simulink subsystem "PWM"  (R2020b)
settings: Solver=VariableStepAuto  StartTime=0.0  StopTime=10.0  RelTol=1e-3
libraries: fl_lib x46, ee_lib x14, nesl_utility x12
settings Model: Creator=marti  LastModifiedBy=marti

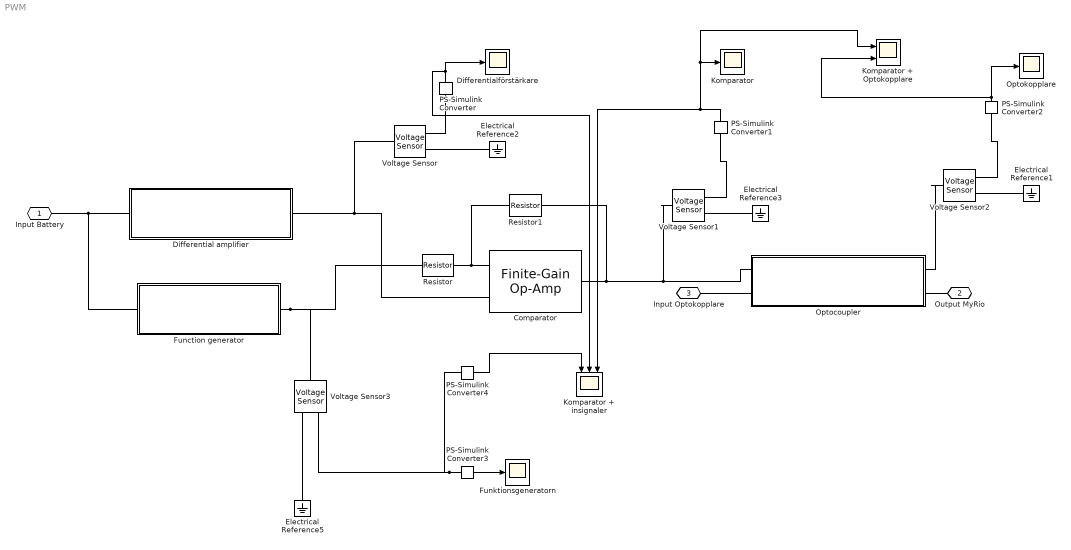
== system PWM ==
  Comparator : ee_lib/Integrated Circuits/Finite-Gain Op-Amp  A=1000  Rin=1e6 Ohm  Rout=0 Ohm  Vmin=0 V  Vmax=12.8 V  noise_mode=0  v_noise=30e-9 V/Hz^0.50000  noise_prm=1  i_noise=0.5e-12 A/Hz^0.50000  ip_noise=0.5e-12 A/Hz^0.50000  in_noise=0.5e-12 A/Hz^0.50000  sample_time=1e-3 s  repeatability=1  auto_seed_v=576828300  auto_seed_ip=423458404  auto_seed_in=610002388  user_seed_v=0  user_seed_ip=0  user_seed_in=0
      settings: SourceProductBaseCode=PS  InternalSimscapePortConfiguration="{\"Bottom\":[],\"Left\":[{\"id\":\"p\",\"label\":\"+\",\"type\":\"foundation.electrical.electrical\"},{\"id\":\"n\",\"label\":\"-\",\"type\":\"foundation.electrical.electrical\"}],\"Right\":[{\"id\":\"out\",\"label\":\"\",\"type\":\"foundation.electrical.electrical\"}],\"Top\":[]}"
  Differential amplifier : Subsystem
  Differentialförstärkare : Scope
  Electrical Reference{1..3,5} (4 alike) : fl_lib/Electrical/Electrical Elements/Electrical Reference
  Function generator : Subsystem
  Funktionsgeneratorn : Scope
  Komparator : Scope
  Komparator + Optokopplare : Scope  NumInputPorts=2
  Komparator + insignaler : Scope  NumInputPorts=3
  Optocoupler : Subsystem
  Optokopplare : Scope
  PS-Simulink Converter : nesl_utility/PS-Simulink Converter  PhysicalDomain=network_engine_domain  SubClassName=ps_output  LeftPortType=input  RightPortType=output  PseudoPeriodic=off  Frequencies=[]  Unit=inherit  AffineConversion=off
  PS-Simulink Converter1 : nesl_utility/PS-Simulink Converter  PhysicalDomain=network_engine_domain  SubClassName=ps_output  LeftPortType=input  RightPortType=output  PseudoPeriodic=off  Frequencies=[]  Unit=inherit  AffineConversion=off
  PS-Simulink Converter2 : nesl_utility/PS-Simulink Converter  PhysicalDomain=network_engine_domain  SubClassName=ps_output  LeftPortType=input  RightPortType=output  PseudoPeriodic=off  Frequencies=[]  Unit=inherit  AffineConversion=off
  PS-Simulink Converter3 : nesl_utility/PS-Simulink Converter  PhysicalDomain=network_engine_domain  SubClassName=ps_output  LeftPortType=input  RightPortType=output  PseudoPeriodic=off  Frequencies=[]  Unit=1  AffineConversion=off
  PS-Simulink Converter4 : nesl_utility/PS-Simulink Converter  PhysicalDomain=network_engine_domain  SubClassName=ps_output  LeftPortType=input  RightPortType=output  PseudoPeriodic=off  Frequencies=[]  Unit=1  AffineConversion=off
  Resistor : fl_lib/Electrical/Electrical Elements/Resistor  R=10000 Ohm  i_specify=off  i_priority=None  i=0 A  i_nominal_specify=off  i_nominal_unit=A  i_nominal_value=1  v_specify=off  v_priority=None  v=0 V  v_nominal_specify=off  v_nominal_unit=V  v_nominal_value=1
  Resistor1 : fl_lib/Electrical/Electrical Elements/Resistor  R=100000 Ohm  i_specify=off  i_priority=None  i=0 A  i_nominal_specify=off  i_nominal_unit=A  i_nominal_value=1  v_specify=off  v_priority=None  v=0 V  v_nominal_specify=off  v_nominal_unit=V  v_nominal_value=1
  Voltage Sensor{,1..3} (4 alike) : fl_lib/Electrical/Electrical Sensors/Voltage Sensor
      Voltage Sensor3 settings: SourceProductName=Foundation Library
      Voltage Sensor settings: LogSimulationData=on
  Input Battery : PMIOPort  Side=Left
  Output MyRio : PMIOPort  Port=2  Side=Right
  Input Optokopplare : PMIOPort  Port=3  Side=Left
  wires:
  PS-Simulink Converter/1 -> Komparator + insignaler/2, Differentialförstärkare/1
  PS-Simulink Converter3/1 -> Funktionsgeneratorn/1
  PS-Simulink Converter4/1 -> Komparator + insignaler/1
  PS-Simulink Converter2/1 -> Komparator + Optokopplare/2, Optokopplare/1
  PS-Simulink Converter1/1 -> Komparator/1, Komparator + Optokopplare/1, Komparator + insignaler/3
  connections:
  Function generator/LConn1 -- Input Battery/RConn1 -- Differential amplifier/LConn1
  PS-Simulink Converter3/LConn1 -- Voltage Sensor3/RConn1 -- PS-Simulink Converter4/LConn1
  Differential amplifier/RConn1 -- Voltage Sensor/LConn1 -- Comparator/LConn2
  Function generator/RConn1 -- Voltage Sensor3/LConn1 -- Resistor/LConn1
  Resistor1/RConn1 -- Comparator/RConn1 -- Voltage Sensor1/LConn1 -- Optocoupler/LConn1
  Resistor1/LConn1 -- Resistor/RConn1 -- Comparator/LConn1
  Input Optokopplare/RConn1 -- Optocoupler/LConn2
  Optocoupler/RConn2 -- Output MyRio/RConn1
  Voltage Sensor/RConn1 -- PS-Simulink Converter/LConn1
  Voltage Sensor3/RConn2 -- Electrical Reference5/LConn1
  Electrical Reference3/LConn1 -- Voltage Sensor1/RConn2
  Voltage Sensor2/LConn1 -- Optocoupler/RConn1
  PS-Simulink Converter1/LConn1 -- Voltage Sensor1/RConn1
  Voltage Sensor/RConn2 -- Electrical Reference2/LConn1
  Electrical Reference1/LConn1 -- Voltage Sensor2/RConn2
  PS-Simulink Converter2/LConn1 -- Voltage Sensor2/RConn1

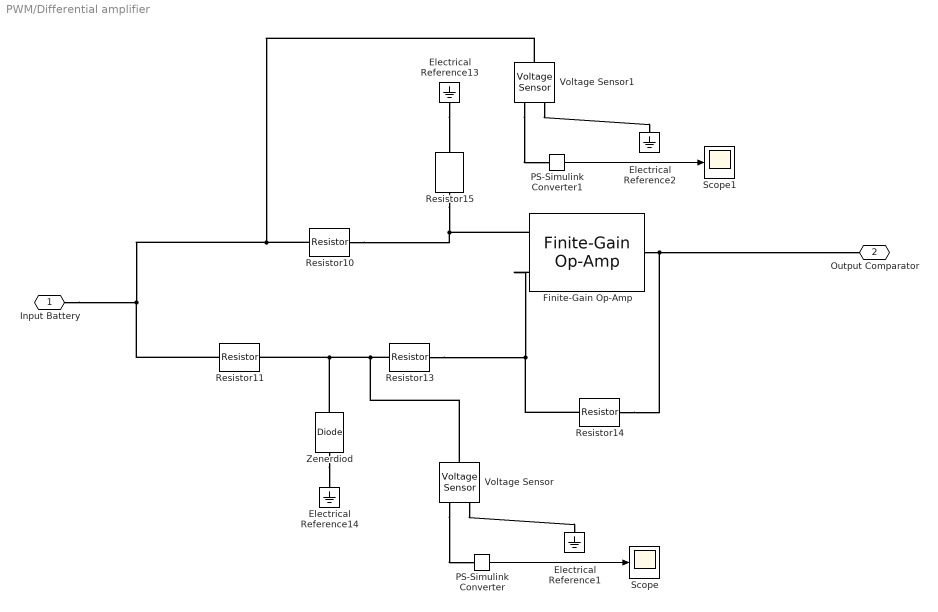
== system PWM/Differential amplifier ==
  Electrical Reference{1..2,13..14} (4 alike) : fl_lib/Electrical/Electrical Elements/Electrical Reference
  Finite-Gain Op-Amp : ee_lib/Integrated Circuits/Finite-Gain Op-Amp  A=1000  Rin=1e6 Ohm  Rout=0 Ohm  Vmin=0 V  Vmax=12.8 V  noise_mode=0  v_noise=30e-9 V/Hz^0.50000  noise_prm=1  i_noise=0.5e-12 A/Hz^0.50000  ip_noise=0.5e-12 A/Hz^0.50000  in_noise=0.5e-12 A/Hz^0.50000  sample_time=1e-3 s  repeatability=1  auto_seed_v=722633825  auto_seed_ip=842882703  auto_seed_in=1363565252  user_seed_v=0  user_seed_ip=0  user_seed_in=0
      settings: SourceProductBaseCode=PS  LogSimulationData=on  InternalSimscapePortConfiguration="{\"Bottom\":[],\"Left\":[{\"id\":\"p\",\"label\":\"+\",\"type\":\"foundation.electrical.electrical\"},{\"id\":\"n\",\"label\":\"-\",\"type\":\"foundation.electrical.electrical\"}],\"Right\":[{\"id\":\"out\",\"label\":\"\",\"type\":\"foundation.electrical.electrical\"}],\"Top\":[]}"
  PS-Simulink Converter : nesl_utility/PS-Simulink Converter  PhysicalDomain=network_engine_domain  SubClassName=ps_output  LeftPortType=input  RightPortType=output  PseudoPeriodic=off  Frequencies=[]  Unit=inherit  AffineConversion=off
  PS-Simulink Converter1 : nesl_utility/PS-Simulink Converter  PhysicalDomain=network_engine_domain  SubClassName=ps_output  LeftPortType=input  RightPortType=output  PseudoPeriodic=off  Frequencies=[]  Unit=inherit  AffineConversion=off
  Resistor10 : fl_lib/Electrical/Electrical Elements/Resistor  R=1000 Ohm  i_specify=off  i_priority=None  i=0 A  i_nominal_specify=off  i_nominal_unit=A  i_nominal_value=1  v_specify=off  v_priority=None  v=0 V  v_nominal_specify=off  v_nominal_unit=V  v_nominal_value=1
  Resistor11 : fl_lib/Electrical/Electrical Elements/Resistor  R=300 Ohm  i_specify=off  i_priority=None  i=0 A  i_nominal_specify=off  i_nominal_unit=A  i_nominal_value=1  v_specify=off  v_priority=None  v=0 V  v_nominal_specify=off  v_nominal_unit=V  v_nominal_value=1
  Resistor13 : fl_lib/Electrical/Electrical Elements/Resistor  R=1000 Ohm  i_specify=off  i_priority=None  i=0 A  i_nominal_specify=off  i_nominal_unit=A  i_nominal_value=1  v_specify=off  v_priority=None  v=0 V  v_nominal_specify=off  v_nominal_unit=V  v_nominal_value=1
  Resistor14 : fl_lib/Electrical/Electrical Elements/Resistor  R=7000 Ohm  i_specify=off  i_priority=None  i=0 A  i_nominal_specify=off  i_nominal_unit=A  i_nominal_value=1  v_specify=off  v_priority=None  v=0 V  v_nominal_specify=off  v_nominal_unit=V  v_nominal_value=1
  Resistor15 : fl_lib/Electrical/Electrical Elements/Resistor  R=7000 Ohm  i_specify=off  i_priority=None  i=0 A  i_nominal_specify=off  i_nominal_unit=A  i_nominal_value=1  v_specify=off  v_priority=None  v=0 V  v_nominal_specify=off  v_nominal_unit=V  v_nominal_value=1
  Scope : Scope
  Scope1 : Scope
  Voltage Sensor : fl_lib/Electrical/Electrical Sensors/Voltage Sensor
  Voltage Sensor1 : fl_lib/Electrical/Electrical Sensors/Voltage Sensor
  Zenerdiod : ee_lib/Semiconductors & Converters/Diode  ModelType=ee.enum.diode.modelType.pwl  IfMat=[.07, .12, .19, 1.75, 4.24, 7.32, 11.2; .16, .3, .72, 2.14, 4.02, 6.35, 9.12] A  TjVec=[25, 125] degC  VfVec=[.5, .7, .9, 1.3, 1.7, 2.1, 2.5] V  Vf=0.6 V  Ron=0.3 Ohm  Goff=1e-8 S  prmExp=ee.enum.diode.expParam.useTwo  I12=[.0137, .545] A  V12=[.6, .7] V  IS=1e-12 A  ec=1  I1=0.0137 A  V1=0.6 V  RS=0 Ohm  Tmeas=25 degC  N_series=1  N_parallel=1  Rz=0.3 Ohm  BV=11.5 V  C_param=ee.enum.diode.capParam.fixed  CJ=5 pF  CJ0=5 pF  VJ=1 V  Mgrad=0.5  Vvec=[.1, 10, 100] V  Cvec=[3.5, 1, .4] pF  FC=0.5  Q_param=ee.enum.diode.recoveryParam.off  iRM=-7.15 A  iF=4 A  didt=-750 A/us  trr_factor=3  trr=115 ns  Qrr=1500 s*uA  TT=50 ns  tau=100 ns  T_param=ee.enum.diode.temperatureParam.off  IS_T2=1.25e-7 A  I1_T2=0.245 A  V1_T2=0.5 V  Tmeas2=125 degC  EG_param=ee.enum.diode.egapParam.material_si  EG=1.11 eV  XTI_param=ee.enum.diode.xtiParam.pn  XTI=3  dBVdT=0 V/K  Tdevice=25 degC  i_specify=off  i_priority=None  i=0 A  i_nominal_specify=off  i_nominal_unit=A  i_nominal_value=1  v_specify=off  v_priority=None  v=0 V  v_nominal_specify=off  v_nominal_unit=V  v_nominal_value=1  i_capacitor_specify=off  i_capacitor_priority=None  i_capacitor=0 A  i_capacitor_nominal_specify=off  i_capacitor_nominal_unit=A  i_capacitor_nominal_value=1  v_capacitor_specify=off  v_capacitor_priority=None  v_capacitor=0 V  v_capacitor_nominal_specify=off  v_capacitor_nominal_unit=V  v_capacitor_nominal_value=1  power_dissipated_specify=off  power_dissipated_priority=None  power_dissipated=0 W  power_dissipated_nominal_specify=off  power_dissipated_nominal_unit=W  power_dissipated_nominal_value=1  thermal_network_parameterization=ee.enum.thermalNetworkTopology.cauer  Rth=[0, 10] K/W  Rth_Foster=[4, 6] K/W  thermal_mass_parameterization=ee.enum.thermalNetwork.timeconstant  thermal_mass=[0, 1] J/K  thermal_mass_Foster=[1.5, 3] J/K  thermal_time_constant=[0, 10] s  thermal_time_constant_Foster=[6, 18] s  thermal_mass_initial_temperatures=[25, 25] degC
  Input Battery : PMIOPort  Side=Left
  Output Comparator : PMIOPort  Port=2  Side=Right
  wires:
  PS-Simulink Converter/1 -> Scope/1
  PS-Simulink Converter1/1 -> Scope1/1
  connections:
  Zenerdiod/LConn1 -- Electrical Reference14/LConn1
  Resistor10/RConn1 -- Finite-Gain Op-Amp/LConn1 -- Resistor15/LConn1
  Resistor11/LConn1 -- Input Battery/RConn1 -- Resistor10/LConn1 -- Voltage Sensor1/LConn1
  Resistor13/RConn1 -- Finite-Gain Op-Amp/LConn2 -- Resistor14/LConn1
  Electrical Reference13/LConn1 -- Resistor15/RConn1
  Resistor13/LConn1 -- Voltage Sensor/LConn1 -- Zenerdiod/RConn1 -- Resistor11/RConn1
  Finite-Gain Op-Amp/RConn1 -- Resistor14/RConn1 -- Output Comparator/RConn1
  Voltage Sensor/RConn2 -- Electrical Reference1/LConn1
  Voltage Sensor/RConn1 -- PS-Simulink Converter/LConn1
  Voltage Sensor1/RConn2 -- Electrical Reference2/LConn1
  Voltage Sensor1/RConn1 -- PS-Simulink Converter1/LConn1

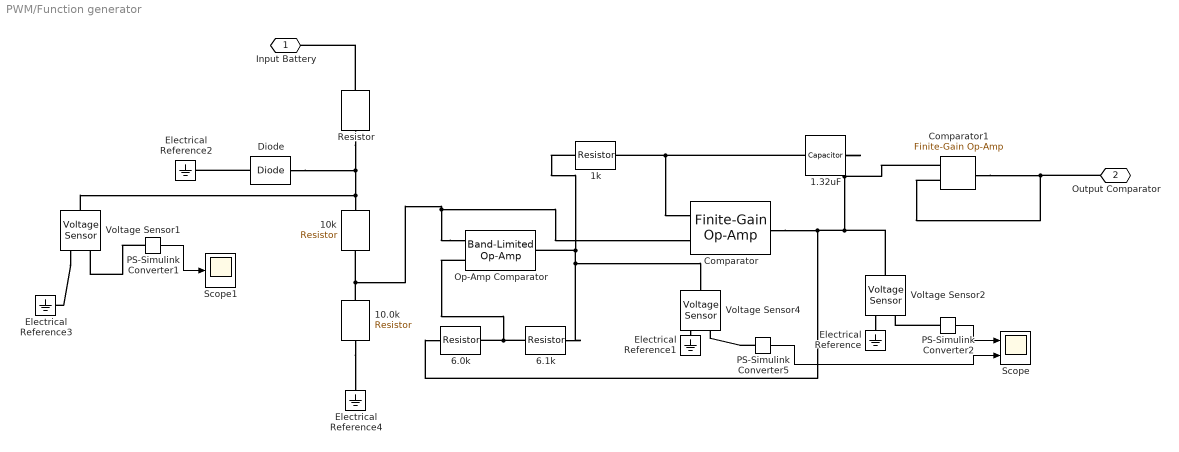
== system PWM/Function generator ==
  1.32uF : ee_lib/Passive/Capacitor  cap_option=0  c=2.64e-6 F  Cvec=[1e-05, 1e-06] F  Vvec=[0, 10] V  CV_table_symmetry=1  f_vec=[1, 10] kHz  DFext_vec=[.8, 1.2]  C_tol=5  enable_C_tol=0  tol_distribution=1  nSigma=4  r=1e-6 Ohm  g=0 1/Ohm  averaging_period=0 s  enable_operating_limits=0  operating_limit_action=2  max_working_voltage_range=[-25, 25] V  power_rating=1 W  enable_faults=0  fault_action=1  Cscale_faulted=100  R_faulted=1e-3 Ohm  G_faulted=0 1/Ohm  tau_fault=1e-3 s  enable_temporal_fault=0  t_fault=1 s  enable_behavioral_fault=0  max_permissible_voltage_range=[-100, 100] V  t_fail_on_voltage=1 s  i_specify=off  i_priority=None  i=0 A  i_nominal_specify=off  i_nominal_unit=A  i_nominal_value=1  v_specify=on  v_priority=None  v=3 V  v_nominal_specify=off  v_nominal_unit=V  v_nominal_value=1  vc_specify=off  vc_priority=High  vc=0 V  vc_nominal_specify=off  vc_nominal_unit=V  vc_nominal_value=1
  10.0k : fl_lib/Electrical/Electrical Elements/Resistor  R=10000 Ohm  i_specify=off  i_priority=None  i=0 A  i_nominal_specify=off  i_nominal_unit=A  i_nominal_value=1  v_specify=off  v_priority=None  v=0 V  v_nominal_specify=off  v_nominal_unit=V  v_nominal_value=1
  10k : fl_lib/Electrical/Electrical Elements/Resistor  R=10000 Ohm  i_specify=off  i_priority=None  i=0 A  i_nominal_specify=off  i_nominal_unit=A  i_nominal_value=1  v_specify=off  v_priority=None  v=0 V  v_nominal_specify=off  v_nominal_unit=V  v_nominal_value=1
  1k : ee_lib/Passive/Resistor  R=1 kOhm  R_tol=5  enable_R_tol=0  tol_distribution=1  nSigma=4  enable_operating_limits=0  operating_limit_action=2  max_working_voltage=100 V  power_rating=1 W  enable_faults=0  fault_action=1  R_faulted=inf Ohm  enable_temporal_fault=0  t_fault=1 s  enable_behavioral_fault=0  max_permissible_current=1 A  t_fail_on_current=1 s  noise_mode=0  sample_time=1e-3 s  repeatability=1  auto_seed=1359052203  user_seed=0  Tdevice=25 degC  alpha=3.93e-3 1/K  Tmeas=25 degC  thermal_mass=100 J/K  power_derating_T1=70 degC  power_derating_T2=155 degC  operating_temperature_range_vec=[-50, 150] degC  temperature_specify=off  temperature_priority=High  temperature=298.15 K  temperature_nominal_specify=off  temperature_nominal_unit=K  temperature_nominal_value=1
  6.0k : ee_lib/Passive/Resistor  R=6 kOhm  R_tol=5  enable_R_tol=0  tol_distribution=1  nSigma=4  enable_operating_limits=0  operating_limit_action=2  max_working_voltage=100 V  power_rating=1 W  enable_faults=0  fault_action=1  R_faulted=inf Ohm  enable_temporal_fault=0  t_fault=1 s  enable_behavioral_fault=0  max_permissible_current=1 A  t_fail_on_current=1 s  noise_mode=0  sample_time=1e-3 s  repeatability=1  auto_seed=934427299  user_seed=0  Tdevice=25 degC  alpha=3.93e-3 1/K  Tmeas=25 degC  thermal_mass=100 J/K  power_derating_T1=70 degC  power_derating_T2=155 degC  operating_temperature_range_vec=[-50, 150] degC  temperature_specify=off  temperature_priority=High  temperature=298.15 K  temperature_nominal_specify=off  temperature_nominal_unit=K  temperature_nominal_value=1
  6.1k : ee_lib/Passive/Resistor  R=6.1 kOhm  R_tol=5  enable_R_tol=0  tol_distribution=1  nSigma=4  enable_operating_limits=0  operating_limit_action=2  max_working_voltage=100 V  power_rating=1 W  enable_faults=0  fault_action=1  R_faulted=inf Ohm  enable_temporal_fault=0  t_fault=1 s  enable_behavioral_fault=0  max_permissible_current=1 A  t_fail_on_current=1 s  noise_mode=0  sample_time=1e-3 s  repeatability=1  auto_seed=1078216519  user_seed=0  Tdevice=25 degC  alpha=3.93e-3 1/K  Tmeas=25 degC  thermal_mass=100 J/K  power_derating_T1=70 degC  power_derating_T2=155 degC  operating_temperature_range_vec=[-50, 150] degC  temperature_specify=off  temperature_priority=High  temperature=298.15 K  temperature_nominal_specify=off  temperature_nominal_unit=K  temperature_nominal_value=1
  Comparator : ee_lib/Integrated Circuits/Finite-Gain Op-Amp  A=10000  Rin=1e6 Ohm  Rout=0 Ohm  Vmin=0 V  Vmax=10 V  noise_mode=0  v_noise=30e-9 V/Hz^0.50000  noise_prm=1  i_noise=0.5e-12 A/Hz^0.50000  ip_noise=0.5e-12 A/Hz^0.50000  in_noise=0.5e-12 A/Hz^0.50000  sample_time=1e-3 s  repeatability=1  auto_seed_v=3835072528  auto_seed_ip=3020320751  auto_seed_in=2386876289  user_seed_v=0  user_seed_ip=0  user_seed_in=0
      settings: SourceProductBaseCode=PS  InternalSimscapePortConfiguration="{\"Bottom\":[],\"Left\":[{\"id\":\"p\",\"label\":\"+\",\"type\":\"foundation.electrical.electrical\"},{\"id\":\"n\",\"label\":\"-\",\"type\":\"foundation.electrical.electrical\"}],\"Right\":[{\"id\":\"out\",\"label\":\"\",\"type\":\"foundation.electrical.electrical\"}],\"Top\":[]}"
  Comparator1 : ee_lib/Integrated Circuits/Finite-Gain Op-Amp  A=1000  Rin=1e6 Ohm  Rout=0 Ohm  Vmin=0 V  Vmax=10 V  noise_mode=0  v_noise=30e-9 V/Hz^0.50000  noise_prm=1  i_noise=0.5e-12 A/Hz^0.50000  ip_noise=0.5e-12 A/Hz^0.50000  in_noise=0.5e-12 A/Hz^0.50000  sample_time=1e-3 s  repeatability=1  auto_seed_v=792136572  auto_seed_ip=910665535  auto_seed_in=332202012  user_seed_v=0  user_seed_ip=0  user_seed_in=0
      settings: SourceProductBaseCode=PS  InternalSimscapePortConfiguration="{\"Bottom\":[],\"Left\":[{\"id\":\"p\",\"label\":\"+\",\"type\":\"foundation.electrical.electrical\"},{\"id\":\"n\",\"label\":\"-\",\"type\":\"foundation.electrical.electrical\"}],\"Right\":[{\"id\":\"out\",\"label\":\"\",\"type\":\"foundation.electrical.electrical\"}],\"Top\":[]}"
  Diode : ee_lib/Semiconductors & Converters/Diode  ModelType=ee.enum.diode.modelType.pwl  IfMat=[.07, .12, .19, 1.75, 4.24, 7.32, 11.2; .16, .3, .72, 2.14, 4.02, 6.35, 9.12] A  TjVec=[25, 125] degC  VfVec=[.5, .7, .9, 1.3, 1.7, 2.1, 2.5] V  Vf=0.6 V  Ron=0.3 Ohm  Goff=1e-8 S  prmExp=ee.enum.diode.expParam.useTwo  I12=[.0137, .545] A  V12=[.6, .7] V  IS=1e-12 A  ec=1  I1=0.0137 A  V1=0.6 V  RS=0 Ohm  Tmeas=25 degC  N_series=1  N_parallel=1  Rz=0.3 Ohm  BV=10 V  C_param=ee.enum.diode.capParam.fixed  CJ=5 pF  CJ0=5 pF  VJ=1 V  Mgrad=0.5  Vvec=[.1, 10, 100] V  Cvec=[3.5, 1, .4] pF  FC=0.5  Q_param=ee.enum.diode.recoveryParam.off  iRM=-7.15 A  iF=4 A  didt=-750 A/us  trr_factor=3  trr=115 ns  Qrr=1500 s*uA  TT=50 ns  tau=100 ns  T_param=ee.enum.diode.temperatureParam.off  IS_T2=1.25e-7 A  I1_T2=0.245 A  V1_T2=0.5 V  Tmeas2=125 degC  EG_param=ee.enum.diode.egapParam.material_si  EG=1.11 eV  XTI_param=ee.enum.diode.xtiParam.pn  XTI=3  dBVdT=0 V/K  Tdevice=25 degC  i_specify=off  i_priority=None  i=0 A  i_nominal_specify=off  i_nominal_unit=A  i_nominal_value=1  v_specify=off  v_priority=None  v=0 V  v_nominal_specify=off  v_nominal_unit=V  v_nominal_value=1  i_capacitor_specify=off  i_capacitor_priority=None  i_capacitor=0 A  i_capacitor_nominal_specify=off  i_capacitor_nominal_unit=A  i_capacitor_nominal_value=1  v_capacitor_specify=off  v_capacitor_priority=None  v_capacitor=0 V  v_capacitor_nominal_specify=off  v_capacitor_nominal_unit=V  v_capacitor_nominal_value=1  power_dissipated_specify=off  power_dissipated_priority=None  power_dissipated=0 W  power_dissipated_nominal_specify=off  power_dissipated_nominal_unit=W  power_dissipated_nominal_value=1  thermal_network_parameterization=ee.enum.thermalNetworkTopology.cauer  Rth=[0, 10] K/W  Rth_Foster=[4, 6] K/W  thermal_mass_parameterization=ee.enum.thermalNetwork.timeconstant  thermal_mass=[0, 1] J/K  thermal_mass_Foster=[1.5, 3] J/K  thermal_time_constant=[0, 10] s  thermal_time_constant_Foster=[6, 18] s  thermal_mass_initial_temperatures=[25, 25] degC
  Electrical Reference{,1..4} (5 alike) : fl_lib/Electrical/Electrical Elements/Electrical Reference
  Op-Amp Comparator : ee_lib/Integrated Circuits/Band-Limited Op-Amp  A=7.1e4  Rin=39e6 Ohm  Rout=0 Ohm  Vmin=0 V  Vmax=10 V  Vdotmax=1.25/1e-6 V/s  f=4e6 Hz  V0=0 V
      settings: SourceProductName=Electrical
  PS-Simulink Converter1 : nesl_utility/PS-Simulink Converter  PhysicalDomain=network_engine_domain  SubClassName=ps_output  LeftPortType=input  RightPortType=output  PseudoPeriodic=off  Frequencies=[]  Unit=1  AffineConversion=off
  PS-Simulink Converter2 : nesl_utility/PS-Simulink Converter  PhysicalDomain=network_engine_domain  SubClassName=ps_output  LeftPortType=input  RightPortType=output  PseudoPeriodic=off  Frequencies=[]  Unit=1  AffineConversion=off
  PS-Simulink Converter5 : nesl_utility/PS-Simulink Converter  PhysicalDomain=network_engine_domain  SubClassName=ps_output  LeftPortType=input  RightPortType=output  PseudoPeriodic=off  Frequencies=[]  Unit=1  AffineConversion=off
  Resistor : fl_lib/Electrical/Electrical Elements/Resistor  R=200 Ohm  i_specify=off  i_priority=None  i=0 A  i_nominal_specify=off  i_nominal_unit=A  i_nominal_value=1  v_specify=off  v_priority=None  v=0 V  v_nominal_specify=off  v_nominal_unit=V  v_nominal_value=1
  Scope : Scope  NumInputPorts=2
  Scope1 : Scope
  Voltage Sensor1 : fl_lib/Electrical/Electrical Sensors/Voltage Sensor
  Voltage Sensor2 : fl_lib/Electrical/Electrical Sensors/Voltage Sensor
  Voltage Sensor4 : fl_lib/Electrical/Electrical Sensors/Voltage Sensor
  Input Battery : PMIOPort  Side=Left
  Output Comparator : PMIOPort  Port=2  Side=Right
  wires:
  PS-Simulink Converter2/1 -> Scope/1
  PS-Simulink Converter5/1 -> Scope/2
  PS-Simulink Converter1/1 -> Scope1/1
  connections:
  1k/RConn1 -- 1.32uF/LConn1 -- Comparator/LConn2
  Op-Amp Comparator/RConn1 -- 6.1k/RConn1 -- Voltage Sensor4/LConn1 -- 1k/LConn1
  PS-Simulink Converter2/LConn1 -- Voltage Sensor2/RConn1
  Voltage Sensor2/LConn1 -- Comparator/RConn1 -- 6.0k/LConn1 -- 1.32uF/RConn1 -- Comparator1/LConn1
  6.1k/LConn1 -- Op-Amp Comparator/LConn1 -- 6.0k/RConn1
  Comparator1/LConn2 -- Output Comparator/RConn1 -- Comparator1/RConn1
  Op-Amp Comparator/LConn2 -- 10k/RConn1 -- 10.0k/LConn1 -- Comparator/LConn1
  Voltage Sensor4/RConn2 -- Electrical Reference1/LConn1
  Voltage Sensor2/RConn2 -- Electrical Reference/LConn1
  10.0k/RConn1 -- Electrical Reference4/LConn1
  PS-Simulink Converter5/LConn1 -- Voltage Sensor4/RConn1
  Diode/RConn1 -- Resistor/RConn1 -- Voltage Sensor1/LConn1 -- 10k/LConn1
  Resistor/LConn1 -- Input Battery/RConn1
  Diode/LConn1 -- Electrical Reference2/LConn1
  PS-Simulink Converter1/LConn1 -- Voltage Sensor1/RConn1
  Voltage Sensor1/RConn2 -- Electrical Reference3/LConn1

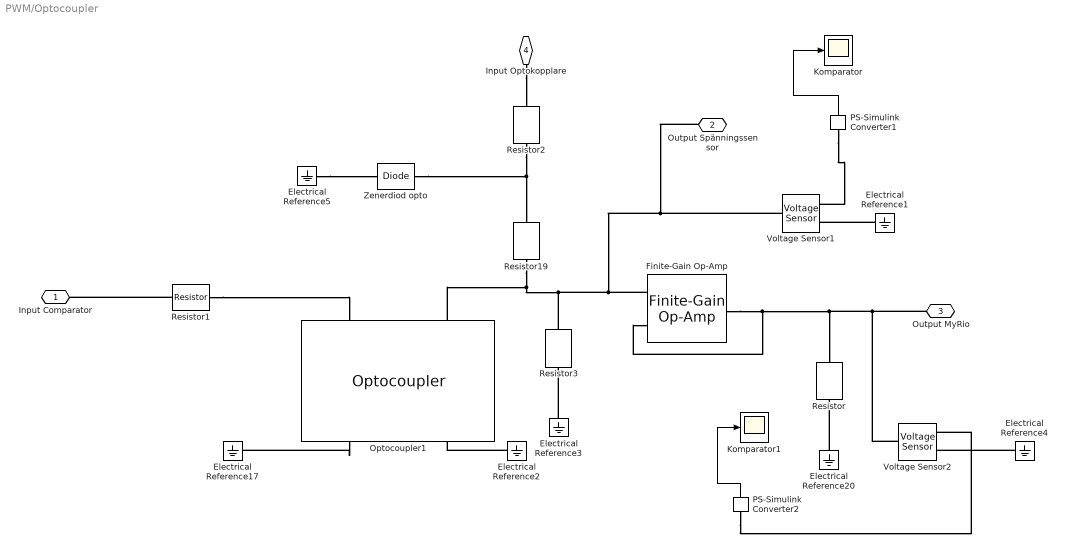
== system PWM/Optocoupler ==
  Electrical Reference{1..5,17,20} (7 alike) : fl_lib/Electrical/Electrical Elements/Electrical Reference
  Finite-Gain Op-Amp : ee_lib/Integrated Circuits/Finite-Gain Op-Amp  A=1000  Rin=1e6 Ohm  Rout=0 Ohm  Vmin=0 V  Vmax=5 V  noise_mode=0  v_noise=30e-9 V/Hz^0.50000  noise_prm=1  i_noise=0.5e-12 A/Hz^0.50000  ip_noise=0.5e-12 A/Hz^0.50000  in_noise=0.5e-12 A/Hz^0.50000  sample_time=1e-3 s  repeatability=1  auto_seed_v=3924742879  auto_seed_ip=3035318747  auto_seed_in=2395685370  user_seed_v=0  user_seed_ip=0  user_seed_in=0
      settings: SourceProductBaseCode=PS  InternalSimscapePortConfiguration="{\"Bottom\":[],\"Left\":[{\"id\":\"p\",\"label\":\"+\",\"type\":\"foundation.electrical.electrical\"},{\"id\":\"n\",\"label\":\"-\",\"type\":\"foundation.electrical.electrical\"}],\"Right\":[{\"id\":\"out\",\"label\":\"\",\"type\":\"foundation.electrical.electrical\"}],\"Top\":[]}"
  Komparator : Scope
  Komparator1 : Scope
  Optocoupler1 : ee_lib/Semiconductors & Converters/Optocoupler  CTR=1  prmExp=1  I12=[.001, .015] A  V12=[.9, 1.05] V  IS=1e-10 A  ec=2  RS=0 Ohm  Tmeas=25 degC  C_param=1  CJ=5 pF  CJ0=5 pF  VJ=1 V  Mgrad=0.5  Vvec=[.1, 10, 100] V  Cvec=[3.5, 1, .4] pF  FC=0.5  T_param=1  IS_T2=1.8e-8 A  I1_T2=0.029 A  V1_T2=1.05 V  Tmeas2=125 degC  EG_param=1  EG=1.11 eV  XTI_param=1  XTI=3  Tdevice=25 degC  i_capacitor_specify=off  i_capacitor_priority=High  i_capacitor=0 A  i_capacitor_nominal_specify=off  i_capacitor_nominal_unit=A  i_capacitor_nominal_value=1  v_capacitor_specify=off  v_capacitor_priority=None  v_capacitor=0 V  v_capacitor_nominal_specify=off  v_capacitor_nominal_unit=V  v_capacitor_nominal_value=1  thermal_network_parameterization=ee.enum.thermalNetworkTopology.cauer  Rth=[0, 10] K/W  Rth_Foster=[4, 6] K/W  thermal_mass_parameterization=ee.enum.thermalNetwork.timeconstant  thermal_mass=[0, 1] J/K  thermal_mass_Foster=[1.5, 3] J/K  thermal_time_constant=[0, 10] s  thermal_time_constant_Foster=[6, 18] s  thermal_mass_initial_temperatures=[25, 25] degC
      settings: SourceProductBaseCode=PS  InternalSimscapePortConfiguration="{\"Bottom\":[],\"Left\":[{\"id\":\"p\",\"label\":\"\",\"type\":\"foundation.electrical.electrical\"},{\"id\":\"C\",\"label\":\"\",\"type\":\"foundation.electrical.electrical\"}],\"Right\":[{\"id\":\"n\",\"label\":\"\",\"type\":\"foundation.electrical.electrical\"},{\"id\":\"E\",\"label\":\"\",\"type\":\"foundation.electrical.electrical\"}],\"Top\":[]}"
  PS-Simulink Converter1 : nesl_utility/PS-Simulink Converter  PhysicalDomain=network_engine_domain  SubClassName=ps_output  LeftPortType=input  RightPortType=output  PseudoPeriodic=off  Frequencies=[]  Unit=inherit  AffineConversion=off
  PS-Simulink Converter2 : nesl_utility/PS-Simulink Converter  PhysicalDomain=network_engine_domain  SubClassName=ps_output  LeftPortType=input  RightPortType=output  PseudoPeriodic=off  Frequencies=[]  Unit=inherit  AffineConversion=off
  Resistor : fl_lib/Electrical/Electrical Elements/Resistor  R=1000 Ohm  i_specify=off  i_priority=None  i=0 A  i_nominal_specify=off  i_nominal_unit=A  i_nominal_value=1  v_specify=off  v_priority=None  v=0 V  v_nominal_specify=off  v_nominal_unit=V  v_nominal_value=1
  Resistor1 : fl_lib/Electrical/Electrical Elements/Resistor  R=720 Ohm  i_specify=off  i_priority=None  i=0 A  i_nominal_specify=off  i_nominal_unit=A  i_nominal_value=1  v_specify=off  v_priority=None  v=0 V  v_nominal_specify=off  v_nominal_unit=V  v_nominal_value=1
  Resistor19 : fl_lib/Electrical/Electrical Elements/Resistor  R=300 Ohm  i_specify=off  i_priority=None  i=0 A  i_nominal_specify=off  i_nominal_unit=A  i_nominal_value=1  v_specify=off  v_priority=None  v=0 V  v_nominal_specify=off  v_nominal_unit=V  v_nominal_value=1
  Resistor2 : fl_lib/Electrical/Electrical Elements/Resistor  R=200 Ohm  i_specify=off  i_priority=None  i=0 A  i_nominal_specify=off  i_nominal_unit=A  i_nominal_value=1  v_specify=off  v_priority=None  v=0 V  v_nominal_specify=off  v_nominal_unit=V  v_nominal_value=1
  Resistor3 : fl_lib/Electrical/Electrical Elements/Resistor  R=1500 Ohm  i_specify=off  i_priority=None  i=0 A  i_nominal_specify=off  i_nominal_unit=A  i_nominal_value=1  v_specify=off  v_priority=None  v=0 V  v_nominal_specify=off  v_nominal_unit=V  v_nominal_value=1
  Voltage Sensor1 : fl_lib/Electrical/Electrical Sensors/Voltage Sensor
  Voltage Sensor2 : fl_lib/Electrical/Electrical Sensors/Voltage Sensor
  Zenerdiod opto : ee_lib/Semiconductors & Converters/Diode  ModelType=ee.enum.diode.modelType.pwl  IfMat=[.07, .12, .19, 1.75, 4.24, 7.32, 11.2; .16, .3, .72, 2.14, 4.02, 6.35, 9.12] A  TjVec=[25, 125] degC  VfVec=[.5, .7, .9, 1.3, 1.7, 2.1, 2.5] V  Vf=0.6 V  Ron=0.3 Ohm  Goff=1e-8 S  prmExp=ee.enum.diode.expParam.useTwo  I12=[.0137, .545] A  V12=[.6, .7] V  IS=1e-12 A  ec=1  I1=0.0137 A  V1=0.6 V  RS=0 Ohm  Tmeas=25 degC  N_series=1  N_parallel=1  Rz=0.3 Ohm  BV=5 V  C_param=ee.enum.diode.capParam.fixed  CJ=5 pF  CJ0=5 pF  VJ=1 V  Mgrad=0.5  Vvec=[.1, 10, 100] V  Cvec=[3.5, 1, .4] pF  FC=0.5  Q_param=ee.enum.diode.recoveryParam.off  iRM=-7.15 A  iF=4 A  didt=-750 A/us  trr_factor=3  trr=115 ns  Qrr=1500 s*uA  TT=50 ns  tau=100 ns  T_param=ee.enum.diode.temperatureParam.off  IS_T2=1.25e-7 A  I1_T2=0.245 A  V1_T2=0.5 V  Tmeas2=125 degC  EG_param=ee.enum.diode.egapParam.material_si  EG=1.11 eV  XTI_param=ee.enum.diode.xtiParam.pn  XTI=3  dBVdT=0 V/K  Tdevice=25 degC  i_specify=off  i_priority=None  i=0 A  i_nominal_specify=off  i_nominal_unit=A  i_nominal_value=1  v_specify=off  v_priority=None  v=0 V  v_nominal_specify=off  v_nominal_unit=V  v_nominal_value=1  i_capacitor_specify=off  i_capacitor_priority=None  i_capacitor=0 A  i_capacitor_nominal_specify=off  i_capacitor_nominal_unit=A  i_capacitor_nominal_value=1  v_capacitor_specify=off  v_capacitor_priority=None  v_capacitor=0 V  v_capacitor_nominal_specify=off  v_capacitor_nominal_unit=V  v_capacitor_nominal_value=1  power_dissipated_specify=off  power_dissipated_priority=None  power_dissipated=0 W  power_dissipated_nominal_specify=off  power_dissipated_nominal_unit=W  power_dissipated_nominal_value=1  thermal_network_parameterization=ee.enum.thermalNetworkTopology.cauer  Rth=[0, 10] K/W  Rth_Foster=[4, 6] K/W  thermal_mass_parameterization=ee.enum.thermalNetwork.timeconstant  thermal_mass=[0, 1] J/K  thermal_mass_Foster=[1.5, 3] J/K  thermal_time_constant=[0, 10] s  thermal_time_constant_Foster=[6, 18] s  thermal_mass_initial_temperatures=[25, 25] degC
  Input Comparator : PMIOPort  Side=Left
  Output Spänningssensor : PMIOPort  Port=2  Side=Right
  Output MyRio : PMIOPort  Port=3  Side=Right
  Input Optokopplare : PMIOPort  Port=4  Side=Left
  wires:
  PS-Simulink Converter1/1 -> Komparator/1
  PS-Simulink Converter2/1 -> Komparator1/1
  connections:
  Optocoupler1/LConn2 -- Output Spänningssensor/RConn1 -- Voltage Sensor1/LConn1 -- Finite-Gain Op-Amp/LConn1 -- Resistor3/LConn1 -- Resistor19/RConn1
  Optocoupler1/RConn1 -- Electrical Reference17/LConn1
  Electrical Reference2/LConn1 -- Optocoupler1/RConn2
  Finite-Gain Op-Amp/LConn2 -- Finite-Gain Op-Amp/RConn1 -- Voltage Sensor2/LConn1 -- Output MyRio/RConn1 -- Resistor/LConn1
  Electrical Reference20/LConn1 -- Resistor/RConn1
  Resistor1/LConn1 -- Input Comparator/RConn1
  Resistor1/RConn1 -- Optocoupler1/LConn1
  Electrical Reference3/LConn1 -- Resistor3/RConn1
  Zenerdiod opto/RConn1 -- Resistor2/RConn1 -- Resistor19/LConn1
  PS-Simulink Converter1/LConn1 -- Voltage Sensor1/RConn1
  Electrical Reference1/LConn1 -- Voltage Sensor1/RConn2
  PS-Simulink Converter2/LConn1 -- Voltage Sensor2/RConn1
  Electrical Reference4/LConn1 -- Voltage Sensor2/RConn2
  Electrical Reference5/LConn1 -- Zenerdiod opto/LConn1
  Input Optokopplare/RConn1 -- Resistor2/LConn1
